simulink model "valve"  (R2019b)
settings: Solver=VariableStepAuto  StartTime=0  StopTime=10  FixedStep=0.001  RelTol=1e-3
undefined symbols (not defined in the file): A_v, C_1, C_2, C_f, gamma, P_0, P_cr, P_s, T
settings Model: Creator=artof  LastModifiedBy=artof

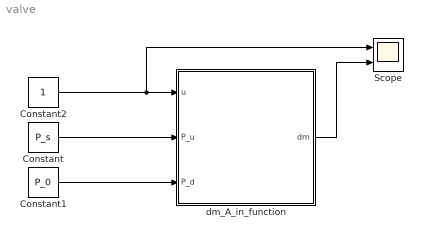
== system valve ==
  Constant : Constant  Value=P_s
  Constant1 : Constant  Value=P_0
  Constant2 : Constant
  Scope : Scope  NumInputPorts=2
  dm_A_in_function : MATLAB Function  TreatAsAtomicUnit=on
  wires:
  dm_A_in_function/1(dm) -> Scope/2
  Constant1/1 -> dm_A_in_function/3(P_d)
  Constant/1 -> dm_A_in_function/2(P_u)
  Constant2/1 -> Scope/1, dm_A_in_function/1(u)

== matlab function valve/dm_A_in_function ==
  data: u input; dm output; P_u input; P_d input; C_f parameter; C_1 parameter; C_2 parameter; P_cr parameter; A_v parameter; T parameter; gamma parameter
function dm = fcn(u, P_u, P_d, C_f, C_1, C_2, P_cr, A_v, T, gamma)
if u > 0    
    P_ratio = P_d/P_u;
    if P_ratio <= P_cr && P_ratio >= 0
        dm = u*C_f*A_v*C_1*P_u/sqrt(T);
    elseif P_ratio > P_cr && P_ratio <= 1
        dm = u*C_f*A_v*C_2*P_u/sqrt(T)*P_ratio^(1/gamma)*sqrt(1-P_ratio^((gamma-1)/gamma));
    else
        %dm = -u*C_f*A_v*C_2*P_d/sqrt(T)*(1/P_ratio)^(1/gamma)*sqrt(1-(1/P_ratio)^((gamma-1)/gamma));
        dm = 0;
    end
else
    dm = 0;
end
